simulink model "whirlybird_sim"  (Simulink 8.5)
settings: Solver=ode45  StartTime=0.0  StopTime=100  RelTol=1e-3
settings Model: Creator=Administrator  LastModifiedBy=jhl48  CovSFcnEnable=off
settings DebuggingCC: SolverPrmCheckMsg=warning  FcnCallInpInsideContextMsg=UseLocalSettings

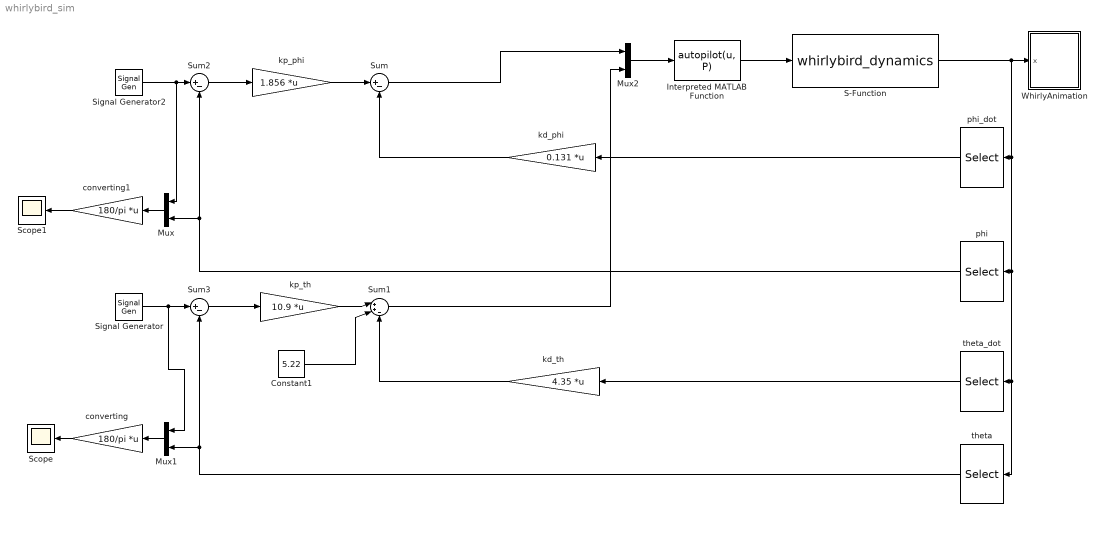
== system whirlybird_sim ==
  Constant1 : Constant  Value=5.22
  Interpreted MATLAB Function : MATLABFcn  MATLABFcn=autopilot(u, P)  OutputDimensions=2  SampleTime=.005
  Mux : Mux  Inputs=2
  Mux1 : Mux  Inputs=2
  Mux2 : Mux  Inputs=2
  S-Function : S-Function  FunctionName=whirlybird_dynamics  Parameters=P
  Scope : Scope
      settings: YMin=-20  YMax=20
  Scope1 : Scope
      settings: YMin=-25  YMax=25
  Signal Generator : SignalGenerator  WaveForm=square  Amplitude=15*pi/180  Frequency=.5  Units=rad/sec
  Signal Generator2 : SignalGenerator  WaveForm=square  Amplitude=20*pi/180*0  Units=rad/sec
  Sum : Sum  Inputs=|+-
  Sum1 : Sum  Inputs=|++-
  Sum2 : Sum  Inputs=|+-
  Sum3 : Sum  Inputs=|+-
  WhirlyAnimation : Subsystem
      mask Display: image(imread('tv.jpg'))
  converting : Gain  Gain=180/pi  Multiplication=Matrix(K*u)
  converting1 : Gain  Gain=180/pi  Multiplication=Matrix(K*u)
  kd_phi : Gain  Gain=0.131  Multiplication=Matrix(K*u)
  kd_th : Gain  Gain=4.35  Multiplication=Matrix(K*u)
  kp_phi : Gain  Gain=1.856  Multiplication=Matrix(K*u)
  kp_th : Gain  Gain=10.9  Multiplication=Matrix(K*u)
  phi : Selector  InputPortWidth=6  Indices=[1]
  phi_dot : Selector  InputPortWidth=6  Indices=[2]
  theta : Selector  InputPortWidth=6  Indices=[3]
  theta_dot : Selector  InputPortWidth=6  Indices=[4]
  wires:
  S-Function/1 -> theta/1, theta_dot/1, phi/1, phi_dot/1, WhirlyAnimation/1(x)
  Interpreted MATLAB Function/1 -> S-Function/1
  phi_dot/1 -> kd_phi/1
  theta_dot/1 -> kd_th/1
  kd_phi/1 -> Sum/2
  kp_th/1 -> Sum1/1
  kp_phi/1 -> Sum/1
  theta/1 -> Mux1/2, Sum3/2
  Sum3/1 -> kp_th/1
  phi/1 -> Mux/2, Sum2/2
  Sum2/1 -> kp_phi/1
  Mux2/1 -> Interpreted MATLAB Function/1
  Sum1/1 -> Mux2/2
  kd_th/1 -> Sum1/3
  Constant1/1 -> Sum1/2
  Mux1/1 -> converting/1
  converting/1 -> Scope/1
  Signal Generator/1 -> Mux1/1, Sum3/1
  converting1/1 -> Scope1/1
  Mux/1 -> converting1/1
  Sum/1 -> Mux2/1
  Signal Generator2/1 -> Mux/1, Sum2/1

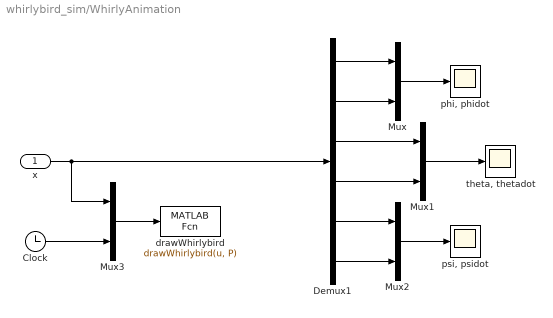
== system whirlybird_sim/WhirlyAnimation ==
  x : Inport
  Clock : Clock
  Demux1 : Demux  Outputs=6
  Mux{,1..3} (4 alike) : Mux  Inputs=2
  drawWhirlybird : MATLABFcn  MATLABFcn=drawWhirlybird(u, P)  OutputDimensions=0  SampleTime=0.1
  "phi, phidot" : Scope
      settings: TimeRange=40  YMin=-10  YMax=15  SaveName=ScopeData4
  "psi, psidot" : Scope
      settings: TimeRange=40  YMin=-2  YMax=1  SaveName=ScopeData3
  "theta, thetadot" : Scope
      settings: TimeRange=40  YMin=-2  YMax=1  SaveName=ScopeData2
  wires:
  Demux1/1 -> Mux/1
  Demux1/2 -> Mux/2
  Demux1/3 -> Mux1/1
  Demux1/4 -> Mux1/2
  Demux1/5 -> Mux2/1
  Demux1/6 -> Mux2/2
  Mux2/1 -> "psi, psidot"/1
  Mux1/1 -> "theta, thetadot"/1
  Mux/1 -> "phi, phidot"/1
  x/1 -> Mux3/1, Demux1/1
  Clock/1 -> Mux3/2
  Mux3/1 -> drawWhirlybird/1
